simulink model "Tp_haxr_mil"  (R2024a)
settings: Solver=ode45  StartTime=0.0  StopTime=0.3  MaxStep=1e-4  RelTol=1e-5
values from neighbouring files (symbols this model uses):
  alpha = 25    [TP_Hacheurs.m]
  E = 0    [TP_Hacheurs.m]
  L = 0.1    [TP_Hacheurs.m]
  R = 10    [TP_Hacheurs.m]
  T = 1/f    (= 0.002)    [TP_Hacheurs.m]
  Vdc = 50    [TP_Hacheurs.m]
libraries: spsDCVoltageSourceLib x3, spsMeanLib x2, spsIGBTDiodeLib x2, spsCurrentMeasurementLib x1, spsSeriesRLCBranchLib x1, spsVoltageMeasurementLib x1, sps_lib x1
settings Model: Creator=Legrey  LastModifiedBy=macbookair
settings RTWCC: GPUComputeCapability=3.5

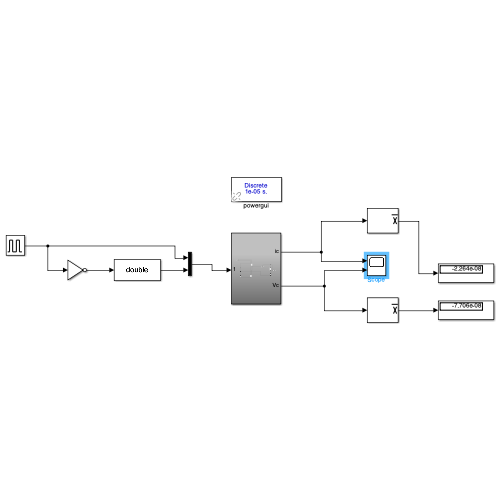
[thumbnail: Simulink's stored preview of the top-level diagram]
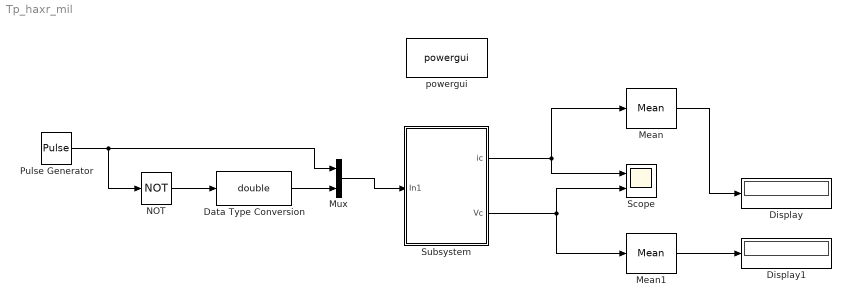
== system Tp_haxr_mil ==
  Data Type Conversion : DataTypeConversion  OutDataTypeStr=double  SaturateOnIntegerOverflow=off  RndMeth=Floor
  Display : Display
  Display1 : Display
  Mean : spsMeanLib/Mean  Freq=f  Vinit=0  Ts=0
  Mean1 : spsMeanLib/Mean  Freq=f  Vinit=0  Ts=0
  Mux : Mux  Inputs=2
  NOT : Logic  Operator=NOT  IconShape=distinctive  AllPortsSameDT=off  OutDataTypeStr=boolean
  Pulse Generator : DiscretePulseGenerator  PulseType=Time based  Period=T  PulseWidth=alpha
  Scope : Scope  NumInputPorts=2
  Subsystem : Subsystem
  powergui : sps_lib/powergui  Priority=1  SimulationMode=Discrete  SampleTime=1e-005  frequency=60  Iterations=50  frequencyindice=0  Pbase=100e6  ErrMax=1e-4  UnitsV=kV  UnitsW=MW  buscounter=0  FunctionMessages=off  echomessages=off  EnableUseOfTLC=off  CurrentSourceSwitches=off  DisableSnubberDevices=off  DisableRonSwitches=off  DisableVfSwitches=off  DisplayEquations=off  AutomaticDiscreteSolvers=off  SolverType=Tustin/Backward Euler (TBE)  Interpol=off  ExternalGateDelay=off  methode=off  Ts=100  x0status=blocks  SPID=on  SwTol=0  HookPort=off  NonlinearTolerance=1e-4  nMaxIteration=100  ContinueOnMaxIteration=off  RestoreLinks=warning  ResistiveCurrentMeasurement=off  Frange=[0:2:500]  Ylog=off  Xlog=on  ShowGrid=off  save=off  variable=ZData  structure=0  ZoomFFT=off  StartTime=0.0  cycles=1  DisplayStyle=1  fundamental=60  FreqAxis=off  MaxFrequency=1000  frequencyindicesteady=1  RmsSteady=1  display=off
  wires:
  Mux/1 -> Subsystem/1(In1)
  Data Type Conversion/1 -> Mux/2
  NOT/1 -> Data Type Conversion/1
  Pulse Generator/1 -> NOT/1, Mux/1
  Subsystem/1(ic) -> Mean/1, Scope/1
  Subsystem/2(Vc) -> Scope/2, Mean1/1
  Mean/1 -> Display/1
  Mean1/1 -> Display1/1

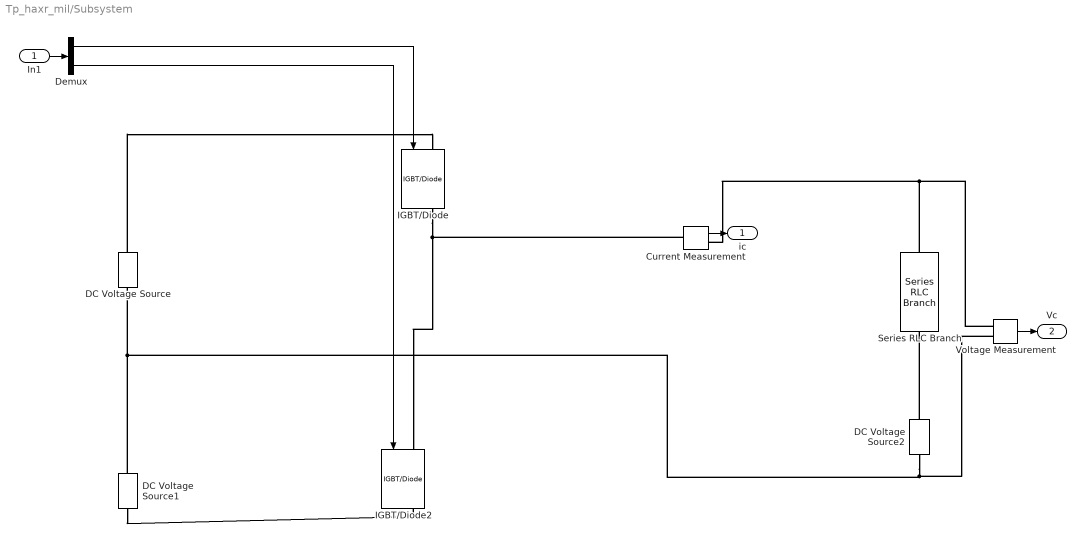
== system Tp_haxr_mil/Subsystem ==
  In1 : Inport
  Current Measurement : spsCurrentMeasurementLib/Current Measurement  PhasorSimulation=off  OutputType=Complex  PSBequivalent=0
  DC Voltage Source : spsDCVoltageSourceLib/DC Voltage Source  Amplitude=Vdc  Measurements=None
  DC Voltage Source1 : spsDCVoltageSourceLib/DC Voltage Source  Amplitude=Vdc  Measurements=None
  DC Voltage Source2 : spsDCVoltageSourceLib/DC Voltage Source  Amplitude=E  Measurements=None
  Demux : Demux  Outputs=2
  IGBT/Diode : spsIGBTDiodeLib/IGBT//Diode  Ron=1e-3  Rs=1e5  Cs=inf  Measurements=on
  IGBT/Diode2 : spsIGBTDiodeLib/IGBT//Diode  Ron=1e-3  Rs=1e5  Cs=inf  Measurements=on
  Series RLC Branch : spsSeriesRLCBranchLib/Series RLC Branch  LConnTagsString=__new0  RConnTagsString=__new0  BranchType=RL  Resistance=R  Inductance=L  SetiL0=off  InitialCurrent=0  Capacitance=1e-6  Setx0=off  InitialVoltage=0  Measurements=None
  Voltage Measurement : spsVoltageMeasurementLib/Voltage Measurement  PhasorSimulation=off  OutputType=Complex  PSBequivalent=0
  ic : Outport
  Vc : Outport  Port=2
  wires:
  Voltage Measurement/1 -> Vc/1
  In1/1 -> Demux/1
  Demux/2 -> IGBT/Diode2/1
  Demux/1 -> IGBT/Diode/1
  Current Measurement/1 -> ic/1
  connections:
  DC Voltage Source/RConn1 -- IGBT/Diode/LConn1
  DC Voltage Source1/RConn1 -- Voltage Measurement/LConn2 -- DC Voltage Source2/LConn1 -- DC Voltage Source/LConn1
  IGBT/Diode/RConn1 -- IGBT/Diode2/LConn1 -- Current Measurement/LConn1
  Series RLC Branch/LConn1 -- Current Measurement/RConn1 -- Voltage Measurement/LConn1
  DC Voltage Source2/RConn1 -- Series RLC Branch/RConn1
  DC Voltage Source1/LConn1 -- IGBT/Diode2/RConn1
